simulink model "Controle_UDP_0809_simulador"  (R2014a)
settings: Solver=ode45  StartTime=0.0  StopTime=360  RelTol=1e-3
values from neighbouring files (symbols this model uses):
  Arwx = [-B1/J1 Kt/J1 ... (first row only)    [data_ACS_HIL.m]
  Arwy = [-B2/J2 Kt/J2 ... (first row only)    [data_ACS_HIL.m]
  Arwz = [-B3/J3 Kt/J3 ... (first row only)    [data_ACS_HIL.m]
  Brwx = [0 ... (first row only)    [data_ACS_HIL.m]
  Brwy = [0 ... (first row only)    [data_ACS_HIL.m]
  Brwz = [0 ... (first row only)    [data_ACS_HIL.m]
  Crwx = [1 0 ... (first row only)    [data_ACS_HIL.m]
  Crwy = [1 0 ... (first row only)    [data_ACS_HIL.m]
  Crwz = [1 0 ... (first row only)    [data_ACS_HIL.m]
  Drwx = zeros(3,1)    [data_ACS_HIL.m]
  Drwy = zeros(3,1)    [data_ACS_HIL.m]
  Drwz = zeros(3,1)    [data_ACS_HIL.m]
  I1 = 0.000624567    [data_ACS_HIL.m]
  I2 = 0.000624567    [data_ACS_HIL.m]
  I3 = 0.000624567    [data_ACS_HIL.m]
  in1 = [ 10 10 25 30 0 ] * pi / 180    [data_ACS_HIL.m]
  in2 = [ 0 10 10 30 0 ] * pi / 180    [data_ACS_HIL.m]
  in3 = [ 45 -30 30 30 0 ] * pi / 180    [data_ACS_HIL.m]
  Ixx = I( 1, 1 )    [data_ACS_HIL.m]
  Iyy = I( 2, 2 )    [data_ACS_HIL.m]
  Izz = I( 3, 3 )    [data_ACS_HIL.m]
  J1 = I1 + 3e-06    (= 0.000627567)    [data_ACS_HIL.m]
  J2 = I2 + 3e-06    (= 0.000627567)    [data_ACS_HIL.m]
  J3 = I3 + 3e-06    (= 0.000627567)    [data_ACS_HIL.m]
  Ki_x = 1    [data_ACS_HIL.m]
  Ki_y = Ki_x    (= 1)    [data_ACS_HIL.m]
  Ki_z = Ki_x    (= 1)    [data_ACS_HIL.m]
  Kp_x = 0.2    [data_ACS_HIL.m]
  Kp_y = Kp_x    (= 0.2)    [data_ACS_HIL.m]
  Kp_z = Kp_x    (= 0.2)    [data_ACS_HIL.m]
  Kpx = vp * (wn^2) * Ixx    [data_ACS_HIL.m]
  Kpy = vp * (wn^2) * Iyy    [data_ACS_HIL.m]
  Kpz = vp * (wn^2) * Izz    [data_ACS_HIL.m]
  Krx = vr * 2 * Ixx * wn * qsi    [data_ACS_HIL.m]
  Kry = vr * 2 * Iyy * wn * qsi    [data_ACS_HIL.m]
  Krz = vr * 2 * Izz * wn * qsi    [data_ACS_HIL.m]
  mW0 = 0000 / ( 60 / ( 2*pi ) )    (= 0)    [data_ACS_HIL.m]
  Wx0 = [mW0 0]    [data_ACS_HIL.m]
  Wy0 = [mW0 0]    [data_ACS_HIL.m]
  Wz0 = [mW0 0]    [data_ACS_HIL.m]
libraries: aerolibconvert2 x6, simulink x6, etargetslib x4, instrumentlib x4, aerolibutil x4, xpcutilitieslib x2, slrtlib x2, rtwinlib x1, aerolibtransform2 x1, vrlib x1
(part 1 of 2)
settings Model: Creator=mayar_000  LastModifiedBy=Toshiba Notebook
settings DataIOCC: SignalLoggingSaveFormat=ModelDataLogs
settings DebuggingCC: MultiTaskDSMMsg=warning  MultiTaskCondExecSysMsg=none  IntegerOverflowMsg=none  ParameterOverflowMsg=none
settings RTWCC: IncludeERTFirstTime=on

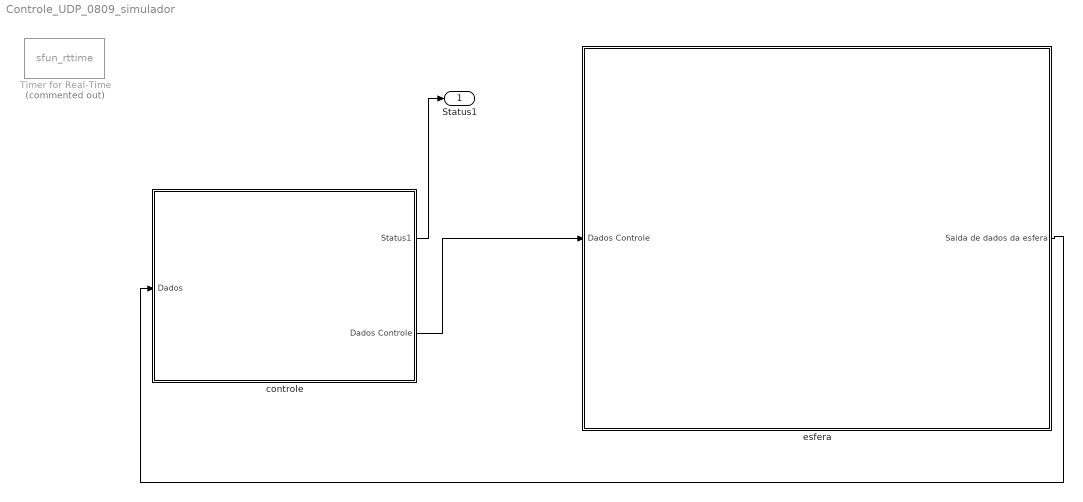
== system Controle_UDP_0809_simulador ==
  Timer for Real-Time : S-Function  Commented=on  FunctionName=sfun_rttime  Parameters=1  EnableBusSupport=off
  "controle " : Subsystem
  "esfera " : Subsystem
  Status1 : Outport
  wires:
  "controle "/1(Status1) -> Status1/1
  "esfera "/1(Saida de dados da esfera) -> "controle "/1(Dados)
  "controle "/2(Dados Controle) -> "esfera "/1(Dados Controle)

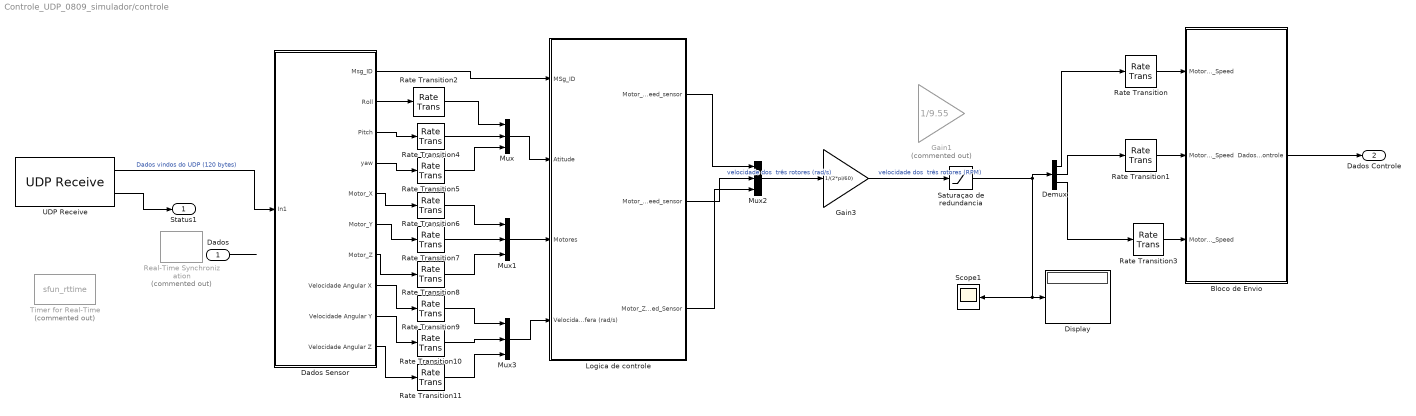
== system Controle_UDP_0809_simulador/controle  ==
  Dados : Inport
  Bloco de Envio : Subsystem
      mask Display:
      | port_label('input',1,'\Omega_x','texmode','on')
      | port_label('input',2,'\Omega_y','texmode','on')
      | port_label('input',3,'\Omega_z','texmode','on')
  Dados Sensor : Subsystem
  Demux : Demux  Outputs=3
  Display : Display
  Gain1 : Gain  Commented=on  Gain=1/9.55  SaturateOnIntegerOverflow=on
  Gain3 : Gain  Gain=1/(2*pi/60)
  Logica de controle : Subsystem
  Mux{,1..3} (4 alike) : Mux  Inputs=3
  Rate Transition{,1..5,9..11} (9 alike) : RateTransition  OutPortSampleTime=t
  Rate Transition6 : RateTransition  X0=5000  OutPortSampleTime=t
  Rate Transition7 : RateTransition  X0=5000  OutPortSampleTime=t
  Rate Transition8 : RateTransition  X0=5000  OutPortSampleTime=t
  Real-Time Synchronization : rtwinlib/Real-Time Synchronization  Commented=on  SampleTime=0.1  MaxMissedTicks=20  ShowMissedTicks=off  YieldWhenWaiting=off
  Saturaçao de redundancia : Saturate  UpperLimit=4000+mW0*60/(2*pi)  LowerLimit=-4000+mW0*60/(2*pi)
  Scope1 : Scope
      settings: YMin=-10000  YMax=10000
  Timer for Real-Time : S-Function  Commented=on  FunctionName=sfun_rttime  Parameters=1  EnableBusSupport=off
  UDP Receive : instrumentlib/UDP Receive  Host=127.0.0.1  Port=35204  LocalPort=35205  DataSize=120  EnableBlockingMode=off  Timeout=50  SampleTime=0.25  DataType=uint8  ByteOrder=BigEndian
  Status1 : Outport
  Dados Controle : Outport  Port=2  OutDataTypeStr=int16
  wires:
  UDP Receive/2 -> Status1/1
  UDP Receive/1 -> Dados Sensor/1(In1)  "Dados vindos do UDP (120 bytes)"
  Rate Transition/1 -> Bloco de Envio/1(Motor_X_Speed)
  Rate Transition1/1 -> Bloco de Envio/2(Motor_Y_Speed)
  Demux/1 -> Rate Transition/1
  Demux/2 -> Rate Transition1/1
  Demux/3 -> Rate Transition3/1
  Rate Transition3/1 -> Bloco de Envio/3(Motor_Z_Speed)
  Dados Sensor/1(Msg_ID) -> Logica de controle/1(MSg_ID)
  Mux/1 -> Logica de controle/2(Atitude)
  Mux1/1 -> Logica de controle/3(Motores)
  Logica de controle/1(Motor_X_Speed_sensor) -> Mux2/1
  Logica de controle/2(Motor_Y_Speed_sensor) -> Mux2/2
  Logica de controle/3(Motor_Z_Speed_Sensor) -> Mux2/3
  Dados Sensor/2(Roll) -> Rate Transition2/1
  Dados Sensor/3(Pitch) -> Rate Transition4/1
  Dados Sensor/4(yaw) -> Rate Transition5/1
  Dados Sensor/7(Motor_Z) -> Rate Transition8/1
  Dados Sensor/6(Motor_Y) -> Rate Transition7/1
  Dados Sensor/5(Motor_X) -> Rate Transition6/1
  Rate Transition2/1 -> Mux/1
  Rate Transition4/1 -> Mux/2
  Rate Transition5/1 -> Mux/3
  Rate Transition6/1 -> Mux1/1
  Rate Transition7/1 -> Mux1/2
  Rate Transition8/1 -> Mux1/3
  Saturaçao de redundancia/1 -> Demux/1, Scope1/1, Display/1
  Mux2/1 -> Gain3/1  "velocidade dos  três rotores (rad/s)"
  Gain3/1 -> Saturaçao de redundancia/1  "velocidade dos  três rotores (RPM)"
  Dados Sensor/8(Velocidade Angular X) -> Rate Transition9/1
  Dados Sensor/9(Velocidade Angular Y) -> Rate Transition10/1
  Dados Sensor/10(Velocidade Angular Z) -> Rate Transition11/1
  Mux3/1 -> Logica de controle/4(Velocidade Angular da Esfera (rad/s))
  Rate Transition9/1 -> Mux3/1
  Rate Transition10/1 -> Mux3/2
  Rate Transition11/1 -> Mux3/3
  Dados/1 -> ?
  Bloco de Envio/1(Dados Controle) -> Dados Controle/1

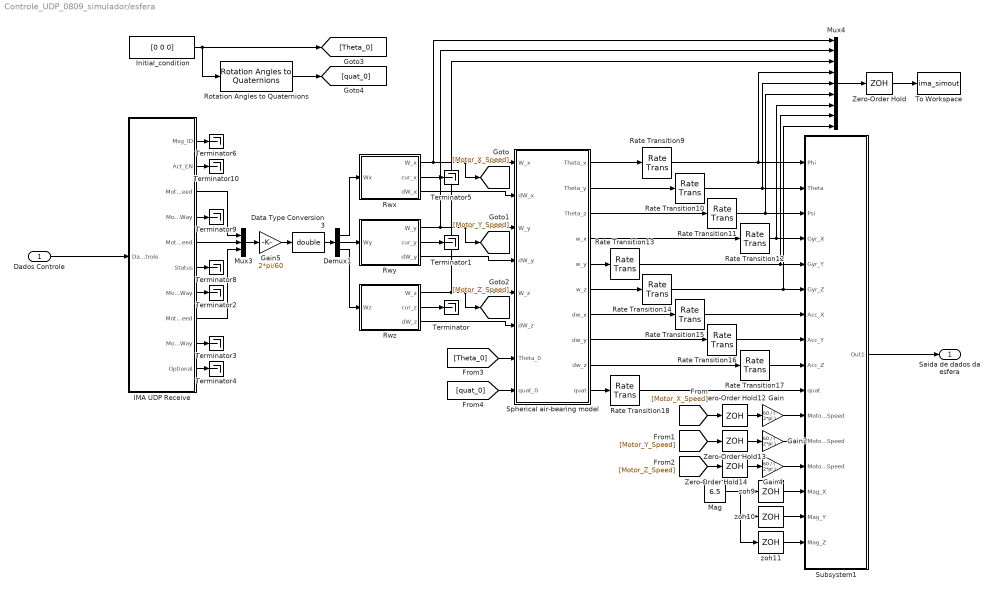
== system Controle_UDP_0809_simulador/esfera  ==
  Dados Controle : Inport
  Data Type Conversion3 : DataTypeConversion  OutDataTypeStr=double  SaturateOnIntegerOverflow=on
  Demux1 : Demux  Outputs=3
  Gain : Gain  Gain=60 / ( 2*pi )
  Gain2 : Gain  Gain=60 / ( 2*pi )
  Gain4 : Gain  Gain=60 / ( 2*pi )
  Gain5 : Gain  Gain=2*pi/60
  IMA UDP Receive : Subsystem
  Initial_condition : Constant  Value=[0 0 0]
  Mag : Constant  Value=6.5  OutDataTypeStr=single
  Mux3 : Mux  Inputs=3
  Mux4 : Mux  Inputs=9
  Rate Transition{9..18} (10 alike) : RateTransition  OutPortSampleTime=t
  Rotation Angles to Quaternions : aerolibtransform2/Rotation Angles to Quaternions  rotationOrder=XYZ
  Rwx : Subsystem
      mask Display:
      | port_label('input',1,'\Omega_{x}^{ref}','texmode','on')
      | 
      | 
      | port_label('output',1,'\Omega_{x}','texmode','on')
      | port_label('output',2,'i_{x}','texmode','on')
      | port_label('output',3,'d\Omega_{x}','texmode','on')
  Rwy : Subsystem
      mask Display:
      | port_label('input',1,'\Omega_{y}^{ref}','texmode','on')
      | 
      | port_label('output',1,'\Omega_{y}','texmode','on')
      | port_label('output',2,'i_{y}','texmode','on')
      | port_label('output',3,'d\Omega_{y}','texmode','on')
  Rwz : Subsystem
      mask Display:
      | port_label('input',1,'\Omega_{z}^{ref}','texmode','on')
      | 
      | port_label('output',1,'\Omega_{z}','texmode','on')
      | port_label('output',2,'i_{z}','texmode','on')
      | port_label('output',3,'d\Omega_{z}','texmode','on')
  Spherical air-bearing model : Subsystem
      mask Display:
      | port_label('input',1,'\Omega_x','texmode','on')
      | port_label('input',2,'d\Omega_x','texmode','on')
      | port_label('input',3,'\Omega_y','texmode','on')
      | port_label('input',4,'d\Omega_y','texmode','on')
      | port_label('input',5,'\Omega_z','texmode','on')
      | port_label('input',6,'d\Omega_z','texmode','on')
      | port_label('input',7,'\theta_{0}','texmode','on')
      | port_label('input',8,'q_{0}','texmode','on')
      | 
      | port_label('output',1,'\theta_x','texmode','on')
      | port_label('output',2,'\theta_y','texmode','on')
      | port_label('output',3,'\theta_z','texmode','on')
      | port_label('output',4,'\omega_x','texmode','on')
      | port_label('output',5,'\omega_y','texmode','on')
      | port_label('output',6,'\omega_z','texmode','on')
      | port_label('output',7,'d\omega_x','texmode','on')
      | port_label('output',8,'d\omega_y','texmode','on')
      | port_label('output',9,'d\omega_z','texmode','on')
      | port_label('output',10,'q','texmode','on')
  Subsystem1 : Subsystem
      mask Display:
      | port_label('input',1,'\theta_x','texmode','on')
      | port_label('input',2,'\theta_y','texmode','on')
      | port_label('input',3,'\theta_z','texmode','on')
      | port_label('input',4,'\omega_x','texmode','on')
      | port_label('input',5,'\omega_y','texmode','on')
      | port_label('input',6,'\omega_z','texmode','on')
      | port_label('input',7,'d\omega_x','texmode','on')
      | port_label('input',8,'d\omega_y','texmode','on')
      | port_label('input',9,'d\omega_z','texmode','on')
      | port_label('input',10,'q','texmode','on')
      | port_label('input',11,'\Omega_x','texmode','on')
      | port_label('input',12,'\Omega_y','texmode','on')
      | port_label('input',13,'\Omega_z','texmode','on')
      | port_label('input',14,'B_x','texmode','on')
      | port_label('input',15,'B_y','texmode','on')
      | port_label('input',16,'B_z','texmode','on')
  Terminator{,1..6,8..10} (10 alike) : Terminator
  To Workspace : ToWorkspace  VariableName=ima_simout  SampleTime=-1
  Zero-Order Hold : ZeroOrderHold  SampleTime=0.5
  Zero-Order Hold12 : ZeroOrderHold  SampleTime=t
  Zero-Order Hold13 : ZeroOrderHold  SampleTime=t
  Zero-Order Hold14 : ZeroOrderHold  SampleTime=t
  zoh10 : ZeroOrderHold  SampleTime=t
  zoh11 : ZeroOrderHold  SampleTime=t
  zoh9 : ZeroOrderHold  SampleTime=t
  Saida de dados da esfera : Outport
  wires:
  Rate Transition12/1 -> Subsystem1/4(Gyr_X), Mux4/7
  Spherical air-bearing model/2(Theta_y) -> Rate Transition10/1
  Initial_condition/1 -> [Theta_0], Rotation Angles to Quaternions/1
  Rwy/2(cur_y) -> Terminator1/1
  Rate Transition16/1 -> Subsystem1/8(Acc_Y)
  IMA UDP Receive/7(Motor_Y_Way) -> Terminator2/1
  IMA UDP Receive/9(Motor_Z_Way) -> Terminator3/1
  Data Type Conversion3/1 -> Demux1/1
  Spherical air-bearing model/4(w_x) -> Rate Transition12/1
  IMA UDP Receive/4(Motor_X_Way) -> Terminator9/1
  Spherical air-bearing model/3(Theta_z) -> Rate Transition11/1
  IMA UDP Receive/5(Motor_Y_Speed) -> Mux3/2
  IMA UDP Receive/10(Optional) -> Terminator4/1
  Rate Transition17/1 -> Subsystem1/9(Acc_Z)
  zoh9/1 -> Subsystem1/14(Mag_X)
  Spherical air-bearing model/6(w_z) -> Rate Transition14/1
  Rate Transition11/1 -> Subsystem1/3(Psi), Mux4/6
  Spherical air-bearing model/8(dw_y) -> Rate Transition16/1
  Rate Transition10/1 -> Subsystem1/2(Theta), Mux4/5
  Spherical air-bearing model/7(dw_x) -> Rate Transition15/1
  Demux1/2 -> Rwy/1(Wy)
  Demux1/3 -> Rwz/1(Wz)
  Rate Transition9/1 -> Subsystem1/1(Phi), Mux4/4
  Rate Transition15/1 -> Subsystem1/7(Acc_X)
  zoh11/1 -> Subsystem1/16(Mag_Z)
  zoh10/1 -> Subsystem1/15(Mag_Y)
  Spherical air-bearing model/9(dw_z) -> Rate Transition17/1
  Rwz/2(cur_z) -> Terminator/1
  IMA UDP Receive/1(Msg_ID) -> Terminator6/1
  IMA UDP Receive/6(Status) -> Terminator8/1
  IMA UDP Receive/2(Act_EN) -> Terminator10/1
  Rate Transition13/1 -> Subsystem1/5(Gyr_Y), Mux4/8
  Demux1/1 -> Rwx/1(Wx)
  Spherical air-bearing model/1(Theta_x) -> Rate Transition9/1
  Rate Transition14/1 -> Subsystem1/6(Gyr_Z), Mux4/9
  Spherical air-bearing model/5(w_y) -> Rate Transition13/1
  [Theta_0] -> Spherical air-bearing model/7(Theta_0)
  Mux3/1 -> Gain5/1
  Spherical air-bearing model/10(quat) -> Rate Transition18/1
  Rwz/1(W_z) -> Spherical air-bearing model/5(W_z), [Motor_Z_Speed], Mux4/3
  Gain/1 -> Subsystem1/11(Motor_X_Speed)
  [Motor_X_Speed] -> Zero-Order Hold12/1
  IMA UDP Receive/8(Motor_Z_Speed) -> Mux3/3
  Zero-Order Hold14/1 -> Gain4/1
  Rwx/2(cur_x) -> Terminator5/1
  IMA UDP Receive/3(Motor_X_Speed) -> Mux3/1
  Gain5/1 -> Data Type Conversion3/1
  Gain2/1 -> Subsystem1/12(Motor_Y_Speed)
  Mag/1 -> zoh9/1, zoh10/1, zoh11/1
  [Motor_Y_Speed] -> Zero-Order Hold13/1
  Gain4/1 -> Subsystem1/13(Motor_Z_Speed)
  [Motor_Z_Speed] -> Zero-Order Hold14/1
  Zero-Order Hold12/1 -> Gain/1
  [quat_0] -> Spherical air-bearing model/8(quat_0)
  Rotation Angles to Quaternions/1 -> [quat_0]
  Zero-Order Hold13/1 -> Gain2/1
  Rwx/1(W_x) -> Spherical air-bearing model/1(W_x), [Motor_X_Speed], Mux4/1
  Rwz/3(dW_z) -> Spherical air-bearing model/6(dW_z)
  Zero-Order Hold/1 -> To Workspace/1
  Rate Transition18/1 -> Subsystem1/10(quat)
  Rwy/1(W_y) -> Spherical air-bearing model/3(W_y), [Motor_Y_Speed], Mux4/2
  Rwx/3(dW_x) -> Spherical air-bearing model/2(dW_x)
  Rwy/3(dW_y) -> Spherical air-bearing model/4(dW_y)
  Mux4/1 -> Zero-Order Hold/1
  Subsystem1/1(Out1) -> Saida de dados da esfera/1
  Dados Controle/1 -> IMA UDP Receive/1(Dados Controle)

== system Controle_UDP_0809_simulador/controle /Bloco de Envio ==
  Motor_X_Speed : Inport
  Motor_Y_Speed : Inport  Port=2
  Motor_Z_Speed : Inport  Port=3
  "Byte Packing " : xpcutilitieslib/Byte Packing   MaskPackedDataType=uint8  MaskUnpackedDataTypes={'uint8','uint8','int16','uint8','int16','uint8','int16','uint8', 'uint8'}  MaskAlignment=1
  Byte Reversal3 : etargetslib/Byte Reversal  numInp=3
  Data Type Conversion17 : DataTypeConversion  OutDataTypeStr=int16  SaturateOnIntegerOverflow=on
  Data Type Conversion2 : DataTypeConversion  OutDataTypeStr=uint8  SaturateOnIntegerOverflow=on
  Data Type Conversion6 : DataTypeConversion  OutDataTypeStr=int16  SaturateOnIntegerOverflow=on
  Data Type Conversion8 : DataTypeConversion  OutDataTypeStr=int16  SaturateOnIntegerOverflow=on
  Display{1..4} (4 alike) : Display
      Display3 settings: Format=hex (Stored Integer)
      Display4 settings: Format=hex (Stored Integer)
  ID1 : Constant  OutDataTypeStr=uint8
  Mux1 : Mux  Inputs=3
  Mux2 : Mux  Inputs=3
  Mux3 : Mux  Inputs=3
  UDP Send1 : instrumentlib/UDP Send  Host=127.0.0.1  Port=35207  LocalPort=35206  EnableBlockingMode=off  ByteOrder=LittleEndian
  Dados Controle : Outport  OutDataTypeStr=int16
  wires:
  Motor_Y_Speed/1 -> Mux3/2, Data Type Conversion8/1
  Data Type Conversion6/1 -> Mux2/1, Byte Reversal3/1
  Motor_X_Speed/1 -> Mux3/1, Data Type Conversion6/1
  "Byte Packing "/1 -> UDP Send1/1, Display2/1
  Data Type Conversion8/1 -> Mux2/2, Byte Reversal3/2
  Data Type Conversion17/1 -> Mux2/3, Byte Reversal3/3
  Byte Reversal3/2 -> Mux1/2, "Byte Packing "/5
  Data Type Conversion2/1 -> "Byte Packing "/9, "Byte Packing "/8, "Byte Packing "/6, "Byte Packing "/4, "Byte Packing "/2, "Byte Packing "/1
  ID1/1 -> Data Type Conversion2/1
  Byte Reversal3/1 -> Mux1/1, "Byte Packing "/3
  Mux3/1 -> Display1/1
  Mux1/1 -> Display4/1
  Byte Reversal3/3 -> Mux1/3, "Byte Packing "/7
  Motor_Z_Speed/1 -> Mux3/3, Data Type Conversion17/1
  Mux2/1 -> Display3/1

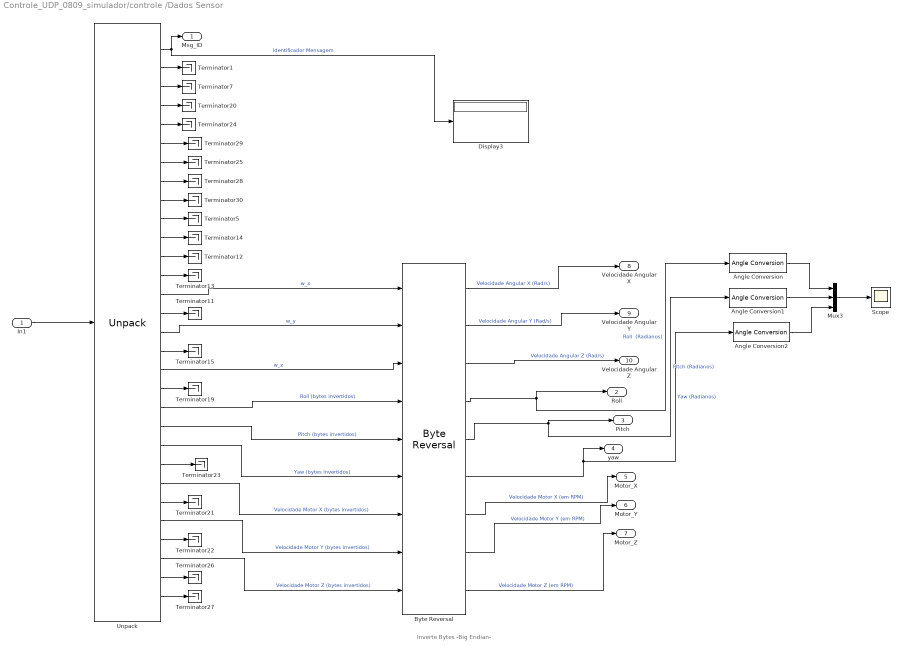
== system Controle_UDP_0809_simulador/controle /Dados Sensor ==
  note: Inverte Bytes
      | -Big Endian-
  In1 : Inport
  Angle Conversion : aerolibconvert2/Angle Conversion  IU=rad  OU=deg
  Angle Conversion1 : aerolibconvert2/Angle Conversion  IU=rad  OU=deg
  Angle Conversion2 : aerolibconvert2/Angle Conversion  IU=rad  OU=deg
  Byte Reversal : etargetslib/Byte Reversal  numInp=9
  Display3 : Display
  Mux3 : Mux  Inputs=3
  Scope : Scope
      settings: YMin=0.2  YMax=1.5  SaveName=ScopeData2
  Terminator{1,5,7,11..15,19..30} (20 alike) : Terminator
  Unpack : slrtlib/UDP/Unpack   dimensions={[1,1],[1,1],[1,1],[1,1],[1,1],[1,1],[1,1],[1,1],[1,1],[1,1],[1,1],[1,1],[1,1],[1,1],[1,1],[1,1],[1,1],[1,1],[1,1],[1,1],[1,1],[1,1],[1,4],[1,1],[1,1],[1,1],[1,1],[1,1],[1,1],[1,1]}  datatypes={'uint8','single','uint32','single','uint32','single','uint32','single','uint32','single','uint32','single','uint32','single','uint32','single','uint32','single','uint32','single','single','single','single','int16','uint32','int16','uint32','int16','uint32','uint8'}  byteAlign=1
  Msg_ID : Outport
  Roll : Outport  Port=2
  Pitch : Outport  Port=3
  yaw : Outport  Port=4
  Motor_X : Outport  Port=5
  Motor_Y : Outport  Port=6
  Motor_Z : Outport  Port=7
  Velocidade Angular X : Outport  Port=8
  Velocidade Angular Y : Outport  Port=9
  Velocidade Angular Z : Outport  Port=10
  wires:
  Unpack/4 -> Terminator20/1
  Unpack/5 -> Terminator24/1
  Unpack/6 -> Terminator29/1
  Unpack/3 -> Terminator7/1
  Byte Reversal/8 -> Motor_Y/1  "Velocidade Motor Y (em RPM)"
  Unpack/1 -> Msg_ID/1, Display3/1  "Identificador Mensagem"
  Unpack/2 -> Terminator1/1
  Unpack/7 -> Terminator25/1
  Unpack/8 -> Terminator28/1
  Byte Reversal/5 -> Pitch/1, Angle Conversion1/1  "Pitch (Radianos)"
  Byte Reversal/7 -> Motor_X/1  "Velocidade Motor X (em RPM)"
  Unpack/28 -> Byte Reversal/9  "Velocidade Motor Z (bytes invertidos)"
  Unpack/19 -> Terminator19/1
  Unpack/11 -> Terminator14/1
  Unpack/14 -> Byte Reversal/1  "w_x"
  Unpack/16 -> Byte Reversal/2  "w_y"
  Unpack/30 -> Terminator27/1
  Unpack/20 -> Byte Reversal/4  "Roll (bytes invertidos)"
  Unpack/21 -> Byte Reversal/5  "Pitch (bytes invertidos)"
  Unpack/12 -> Terminator12/1
  Unpack/23 -> Terminator23/1
  Unpack/18 -> Byte Reversal/3  "w_z"
  Unpack/27 -> Terminator22/1
  Unpack/25 -> Terminator21/1
  Unpack/15 -> Terminator11/1
  Unpack/13 -> Terminator13/1
  Unpack/10 -> Terminator5/1
  Unpack/9 -> Terminator30/1
  Unpack/17 -> Terminator15/1
  Unpack/22 -> Byte Reversal/6  "Yaw (bytes invertidos)"
  Unpack/24 -> Byte Reversal/7  "Velocidade Motor X (bytes invertidos)"
  Unpack/26 -> Byte Reversal/8  "Velocidade Motor Y (bytes invertidos)"
  Unpack/29 -> Terminator26/1
  Byte Reversal/4 -> Roll/1, Angle Conversion/1  "Roll  (Radianos)"
  Byte Reversal/9 -> Motor_Z/1  "Velocidade Motor Z (em RPM)"
  Byte Reversal/6 -> yaw/1, Angle Conversion2/1  "Yaw (Radianos)"
  In1/1 -> Unpack/1
  Angle Conversion/1 -> Mux3/1
  Angle Conversion1/1 -> Mux3/2
  Angle Conversion2/1 -> Mux3/3
  Mux3/1 -> Scope/1
  Byte Reversal/3 -> Velocidade Angular Z/1  "Velocidade Angular Z (Rad/s)"
  Byte Reversal/2 -> Velocidade Angular Y/1  "Velocidade Angular Y (Rad/s)"
  Byte Reversal/1 -> Velocidade Angular X/1  "Velocidade Angular X (Rad/s)"

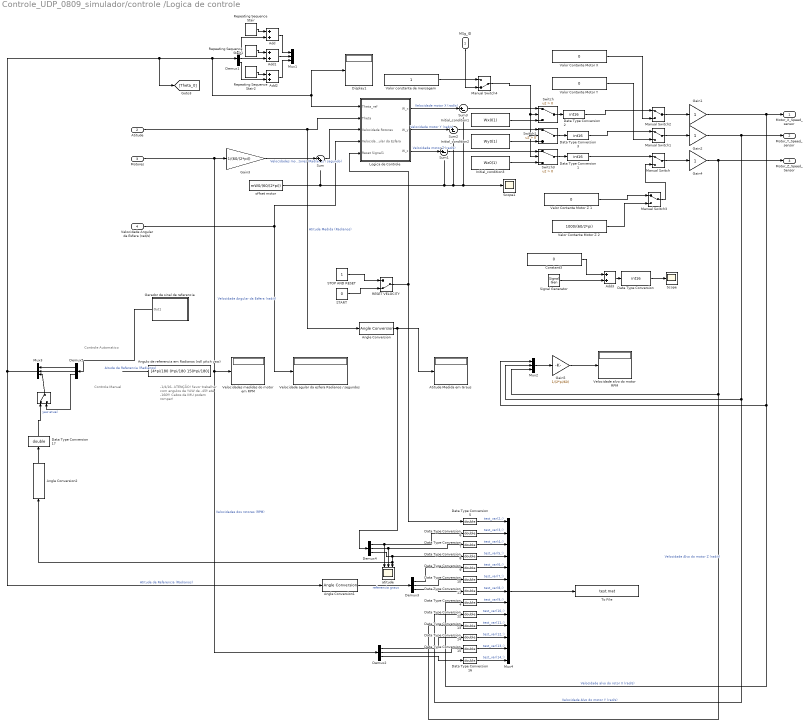
== system Controle_UDP_0809_simulador/controle /Logica de controle ==
  note: Controle Automatico
  note: Controle Manual
  note: -1/4/16-
      | ATENÇÃO!
      |
      | favor trabalhar com
      | angulos de YAW de
      | -45º até -160º!
      | Cabos da IMU podem romper!
  MSg_ID : Inport
  Atitude : Inport  Port=2
  Motores : Inport  Port=3
  Velocidade Angular da Esfera (rad/s) : Inport  Port=4
  " " : ManualSwitch
  Add{,1..3} (4 alike) : Sum
  Angle Conversion : aerolibconvert2/Angle Conversion  IU=rad  OU=deg
  Angle Conversion1 : aerolibconvert2/Angle Conversion  IU=rad  OU=deg
  Angle Conversion2 : aerolibconvert2/Angle Conversion  IU=deg  OU=rad
  Angulo de referencia em Radianos (roll pitch yaw) : Constant  Value=[4*pi/180 0*pi/180 150*pi/180]  VectorParams1D=off
  Atitude Medida em Graus : Display
      settings: Decimation=3
  Constant3 : Constant  Value=0  OutDataTypeStr=int16
  Data Type Conversion : DataTypeConversion  OutDataTypeStr=int16
  Data Type Conversion1 : DataTypeConversion  OutDataTypeStr=int16  SaturateOnIntegerOverflow=on
  Data Type Conversion{4..17} (14 alike) : DataTypeConversion  OutDataTypeStr=double  SaturateOnIntegerOverflow=on
  Data Type Conversion2 : DataTypeConversion  OutDataTypeStr=int16  SaturateOnIntegerOverflow=on
  Data Type Conversion3 : DataTypeConversion  OutDataTypeStr=int16  SaturateOnIntegerOverflow=on
  Demux{1..5} (5 alike) : Demux  Outputs=3
  Display1 : Display
  Gain1 : Gain  OutDataTypeStr=int16  SaturateOnIntegerOverflow=on
  Gain2 : Gain  OutDataTypeStr=int16  SaturateOnIntegerOverflow=on
  Gain3 : Gain  Gain=1/(60/(2*pi))
  Gain4 : Gain  OutDataTypeStr=int16  SaturateOnIntegerOverflow=on
  Gain5 : Gain  Gain=1/(2*pi/60)  OutDataTypeStr=int16  SaturateOnIntegerOverflow=on
  Gerador de sinal de referencia : Subsystem
  Initial_condition1 : Constant  Value=Wx0(1)  OutDataTypeStr=int16
  Initial_condition2 : Constant  Value=Wy0(1)  OutDataTypeStr=int16
  Initial_condition3 : Constant  Value=Wz0(1)  OutDataTypeStr=int16
  Logica de Controle : Subsystem
      mask Display:
      | port_label('input',1,'\theta^{ref}','texmode','on')
      | port_label('input',2,'\theta','texmode','on')
      | port_label('input',3,'\Omega','texmode','on')
      | port_label('input',4,'\omega','texmode','on')
      | port_label('input',5,'RESET','texmode','on')
      | 
      | port_label('output',1,'\Omega_{x}^{des}','texmode','on')
      | port_label('output',2,'\Omega_{y}^{des}','texmode','on')
      | port_label('output',3,'\Omega_{z}^{des}','texmode','on')
  Manual Switch{,1..3} (4 alike) : ManualSwitch
  Manual Switch4 : ManualSwitch  CurrentSetting=0
  Mux1 : Mux  Inputs=3
  Mux2 : Mux  Inputs=3
  Mux3 : Mux  Inputs=3
  Mux4 : Mux  Inputs=13
  RESET VELOCITY : ManualSwitch  CurrentSetting=0
  Repeating Sequence Stair : simulink/Sources/Repeating Sequence Stair  OutValues=in1.'  tsamp=1000  OutMin=[]  OutMax=[]  OutDataTypeStr=double  OutputDataTypeScalingMode=double  OutDataType=fixdt(0,8)  ConRadixGroup=Best Precision: Vector-wise  OutScaling=2^-12
  Repeating Sequence Stair1 : simulink/Sources/Repeating Sequence Stair  OutValues=in2.'  tsamp=1000  OutMin=[]  OutMax=[]  OutDataTypeStr=double  OutputDataTypeScalingMode=double  OutDataType=fixdt(0,8)  ConRadixGroup=Best Precision: Vector-wise  OutScaling=2^-12
  Repeating Sequence Stair2 : simulink/Sources/Repeating Sequence Stair  OutValues=in3.'  tsamp=1000  OutMin=[]  OutMax=[]  OutDataTypeStr=double  OutputDataTypeScalingMode=double  OutDataType=fixdt(0,8)  ConRadixGroup=Best Precision: Vector-wise  OutScaling=2^-12
  START : Constant  Value=0  OutDataTypeStr=boolean
  STOP AND RESET : Constant  OutDataTypeStr=boolean
  Scope : Scope
      settings: YMin=-1050  YMax=-950  SaveName=sinal_referencia
  Scope1 : Scope
      settings: YMin=523.599  YMax=523.599  SaveName=sinal_referencia1
  Signal Generator : SignalGenerator  WaveForm=square  Amplitude=1000  Frequency=0.1
  Sum : Sum  Inputs=|++
  Sum1 : Sum  Inputs=|+-
  Sum2 : Sum  Inputs=|+-
  Sum3 : Sum  Inputs=|+-
  Switch : Switch  Criteria=u2 > Threshold  OutDataTypeStr=int16
  Switch1 : Switch  Criteria=u2 > Threshold  OutDataTypeStr=int16
  Switch3 : Switch  Criteria=u2 > Threshold  OutDataTypeStr=int16
  To File : ToFile  Filename=test.mat  MatrixName=test_var
  Valor Contante Motor X : Constant  Value=0  OutDataTypeStr=int16
  Valor Contante Motor Y : Constant  Value=0  OutDataTypeStr=int16
  Valor Contante Motor Z 1 : Constant  Value=0  OutDataTypeStr=int16
  Valor Contante Motor Z 2 : Constant  Value=1000/(60/2*pi)  OutDataTypeStr=int16
  Valor constante de mensagem : Constant  OutDataTypeStr=int16
  Velocidade agular da esfera Radianos / segundos : Display
      settings: Format=decimal (Stored Integer)  Decimation=3
  Velocidade alvo do motor RPM : Display
      settings: Decimation=3
  Velocidades medidas do motor em RPM : Display
      settings: Decimation=3
  atitude : Scope  NumInputPorts=3
      settings: YMin=3.86202~0.75~-0.5  YMax=3.86202~3~2.25  SaveName=ScopeData4
  offset motor : Constant  Value=mW0/(60/(2*pi))  OutDataTypeStr=double
  Motor_X_Speed_sensor : Outport
  Motor_Y_Speed_sensor : Outport  Port=2
  Motor_Z_Speed_Sensor : Outport  Port=3  OutDataTypeStr=int16
  wires:
  Add1/1 -> Mux1/2
  Demux1/1 -> Add/2
  Add2/1 -> Mux1/3
  Mux3/1 -> Logica de Controle/1(Theta_ref), Display1/1, Demux1/1, [Theta_0], Angle Conversion1/1  "Atitude de Referencia (Radianos)"
  Demux1/2 -> Add1/2
  Repeating Sequence Stair/1 -> Add/1
  Repeating Sequence Stair2/1 -> Add2/1
  Repeating Sequence Stair1/1 -> Add1/1
  Demux1/3 -> Add2/2
  Add/1 -> Mux1/1
  Initial_condition1/1 -> Switch/3
  Motores/1 -> Demux2/1, Velocidades medidas do motor em RPM/1, Gain3/1  "Velocidades dos rotores (RPM)"
  Initial_condition2/1 -> Switch1/3
  Logica de Controle/1(W_x) -> Sum3/1  "Velocidade motor X (rad/s)"
  Logica de Controle/2(W_y) -> Sum2/1  "Velocidade motor Y (rad/s)"
  Logica de Controle/3(W_z) -> Sum1/1  "Velocidade motor Z (rad/s)"
  Switch/1 -> Data Type Conversion2/1
  Data Type Conversion/1 -> Scope/1
  Initial_condition3/1 -> Switch3/3
  Signal Generator/1 -> Add3/2
  Constant3/1 -> Add3/1
  Add3/1 -> Data Type Conversion/1
  Switch3/1 -> Data Type Conversion1/1
  Switch1/1 -> Data Type Conversion3/1
  Valor Contante Motor Y/1 -> Manual Switch1/2
  Valor Contante Motor X/1 -> Manual Switch2/2
  Gain3/1 -> Sum/1  "Velocidades motores (Radianos / segundo)"
  Manual Switch/1 -> Gain4/1
  Manual Switch1/1 -> Gain2/1
  Manual Switch2/1 -> Gain1/1
  Gain1/1 -> Data Type Conversion4/1, Mux2/1, Motor_X_Speed_sensor/1  "Velocidade alvo do rotor X (rad/s)"
  Gain2/1 -> Mux2/2, Data Type Conversion12/1, Motor_Y_Speed_sensor/1  "Velocidade Alvo do motor Y (rad/s)"
  Gain4/1 -> Data Type Conversion13/1, Mux2/3, Motor_Z_Speed_Sensor/1  "Velocidade Alvo do motor Z (rad/s)"
  Atitude/1 -> Logica de Controle/2(Theta), Angle Conversion/1  "Atitude Medida (Radianos)"
  Valor Contante Motor Z 1/1 -> Manual Switch3/1
  Valor Contante Motor Z 2/1 -> Manual Switch3/2
  Manual Switch3/1 -> Manual Switch/2
  Valor constante de mensagem/1 -> Manual Switch4/1
  MSg_ID/1 -> Manual Switch4/2
  Manual Switch4/1 -> Switch3/2, Switch1/2, Switch/2
  STOP AND RESET/1 -> RESET VELOCITY/1
  START/1 -> RESET VELOCITY/2
  Mux2/1 -> Gain5/1
  Gain5/1 -> Velocidade alvo do motor RPM/1
  Sum/1 -> Logica de Controle/3(Velocidade Rotores)
  Velocidade Angular da Esfera (rad/s)/1 -> Logica de Controle/4(Velocidade Angular da Esfera), Velocidade agular da esfera Radianos / segundos/1  "Velocidade Angular da Esfera (rad/s)"
  Angle Conversion/1 -> Demux4/1, Atitude Medida em Graus/1
  Mux4/1 -> To File/1
  RESET VELOCITY/1 -> Data Type Conversion5/1, Logica de Controle/5(Reset Signal1)
  Demux4/2 -> Data Type Conversion7/1, atitude/2
  Demux4/1 -> Data Type Conversion6/1, atitude/1
  Data Type Conversion5/1 -> Mux4/1  "test_var(2,:)"
  Data Type Conversion6/1 -> Mux4/2  "test_var(3,:)"
  Data Type Conversion7/1 -> Mux4/3  "test_var(4,:)"
  Data Type Conversion8/1 -> Mux4/4  "test_var(5,:)"
  Data Type Conversion9/1 -> Mux4/5  "test_var(6,:)"
  Data Type Conversion10/1 -> Mux4/6  "test_var(7,:)"
  Data Type Conversion11/1 -> Mux4/7  "test_var(8,:)"
  Data Type Conversion4/1 -> Mux4/8  "test_var(9,:)"
  Data Type Conversion14/1 -> Mux4/11  "test_var(12,:)"
  Data Type Conversion15/1 -> Mux4/12  "test_var(13,:)"
  Data Type Conversion13/1 -> Mux4/10  "test_var(11,:)"
  Data Type Conversion12/1 -> Mux4/9  "test_var(10,:)"
  Data Type Conversion16/1 -> Mux4/13  "test_var(14,:)"
  Demux2/3 -> Data Type Conversion16/1
  Demux2/1 -> Data Type Conversion14/1
  Demux2/2 -> Data Type Conversion15/1
  Demux3/3 -> Data Type Conversion11/1
  Demux3/2 -> Data Type Conversion10/1
  Demux3/1 -> Data Type Conversion9/1
  Angle Conversion1/1 -> Demux3/1  "referencia graus"
  Demux5/1 -> Mux3/1
  Demux5/2 -> Mux3/2
  Demux4/3 -> Data Type Conversion8/1, Angle Conversion2/1, atitude/3
  Data Type Conversion17/1 -> " "/1  "yaw atual"
  " "/1 -> Mux3/3
  Demux5/3 -> " "/2
  Angle Conversion2/1 -> Data Type Conversion17/1
  Gerador de sinal de referencia/1(Out1) -> Demux5/1
  Angulo de referencia em Radianos (roll pitch yaw)/1 -> ?  "Aitude de Referencia (Radianos)"
  Sum3/1 -> Switch/1
  Sum2/1 -> Switch1/1
  Sum1/1 -> Switch3/1
  Data Type Conversion1/1 -> Manual Switch/1
  Data Type Conversion3/1 -> Manual Switch1/1
  Data Type Conversion2/1 -> Manual Switch2/1
  offset motor/1 -> Scope1/1

== system Controle_UDP_0809_simulador/esfera /IMA UDP Receive ==
  Dados Controle : Inport
  Byte Reversal : etargetslib/Byte Reversal  numInp=3
  Initial_condition : Constant  Value=Wx0(1) * 60 / ( 2*pi )
  Initial_condition1 : Constant  Value=Wy0(1) * 60 / ( 2*pi )
  Initial_condition2 : Constant  Value=Wz0(1) * 60 / ( 2*pi )
  Switch : Switch  Criteria=u2 > Threshold
  Switch1 : Switch  Criteria=u2 > Threshold
  Switch2 : Switch  Criteria=u2 > Threshold
  UDP Receive : instrumentlib/UDP Receive  Host=127.0.0.1  Port=35206  LocalPort=35207  DataSize=12  EnableBlockingMode=off  Timeout=50  SampleTime=0.25  DataType=uint8  ByteOrder=BigEndian
  Unpack1 : slrtlib/UDP/Unpack   dimensions={[1,1],[1,1],[1,1],[1,1],[1,1],[1,1],[1,1],[1,1],[1,1]}  datatypes={'uint8','uint8','int16','uint8','int16','uint8','int16','uint8', 'uint8'}  byteAlign=1
  Msg_ID : Outport
  Act_EN : Outport  Port=2
  Motor_X_Speed : Outport  Port=3
  Motor_X_Way : Outport  Port=4
  Motor_Y_Speed : Outport  Port=5
  Status : Outport  Port=6
  Motor_Y_Way : Outport  Port=7
  Motor_Z_Speed : Outport  Port=8
  Motor_Z_Way : Outport  Port=9
  Optional : Outport  Port=10
  wires:
  Unpack1/9 -> Optional/1
  Unpack1/8 -> Motor_Z_Way/1
  Unpack1/6 -> Motor_Y_Way/1
  Unpack1/4 -> Motor_X_Way/1
  Unpack1/2 -> Act_EN/1
  Unpack1/1 -> Msg_ID/1, Switch1/2, Switch2/2, Switch/2
  Unpack1/3 -> Byte Reversal/1
  Unpack1/5 -> Byte Reversal/2
  Unpack1/7 -> Byte Reversal/3
  UDP Receive/2 -> Status/1
  UDP Receive/1 -> Unpack1/1
  Initial_condition/1 -> Switch/3
  Switch/1 -> Motor_X_Speed/1
  Initial_condition1/1 -> Switch1/3
  Switch1/1 -> Motor_Y_Speed/1
  Initial_condition2/1 -> Switch2/3
  Switch2/1 -> Motor_Z_Speed/1
  Byte Reversal/3 -> Switch2/1
  Byte Reversal/2 -> Switch1/1
  Byte Reversal/1 -> Switch/1
  Dados Controle/1 -> ?

== system Controle_UDP_0809_simulador/esfera /Rwx ==
  Wx : Inport
  Demux : Demux  Outputs=3
  Integrator : Integrator  InitialCondition=Wx0(1)/47.149
  Ki_x : Gain  Gain=Ki_x
  Kp_x : Gain  Gain=Kp_x
  Motor_Rwx : StateSpace  A=Arwx  B=Brwx  C=Crwx  D=Drwx  X0=Wx0
  Saturation : Saturate  UpperLimit=100  LowerLimit=-100
  Sum : Sum  Inputs=|+-
  Sum1 : Sum  Inputs=|++
  W_x : Outport
  cur_x : Outport  Port=2
  dW_x : Outport  Port=3
  wires:
  Sum/1 -> Kp_x/1, Ki_x/1
  Ki_x/1 -> Integrator/1
  Integrator/1 -> Sum1/2
  Kp_x/1 -> Sum1/1
  Sum1/1 -> Saturation/1
  Motor_Rwx/1 -> Demux/1
  Demux/3 -> dW_x/1
  Demux/1 -> Sum/2, W_x/1
  Saturation/1 -> Motor_Rwx/1
  Demux/2 -> cur_x/1
  Wx/1 -> Sum/1

== system Controle_UDP_0809_simulador/esfera /Rwy ==
  Wy : Inport
  Demux : Demux  Outputs=3
  Integrator : Integrator  InitialCondition=Wy0(1)/47.149
  Ki_y : Gain  Gain=Ki_y
  Kp_y : Gain  Gain=Kp_y
  Motor_Rwy : StateSpace  A=Arwy  B=Brwy  C=Crwy  D=Drwy  X0=Wy0
  Saturation : Saturate  UpperLimit=100  LowerLimit=-100
  Sum : Sum  Inputs=|+-
  Sum1 : Sum  Inputs=|++
  W_y : Outport
  cur_y : Outport  Port=2
  dW_y : Outport  Port=3
  wires:
  Sum/1 -> Ki_y/1, Kp_y/1
  Ki_y/1 -> Integrator/1
  Integrator/1 -> Sum1/2
  Kp_y/1 -> Sum1/1
  Sum1/1 -> Saturation/1
  Motor_Rwy/1 -> Demux/1
  Demux/1 -> Sum/2, W_y/1
  Saturation/1 -> Motor_Rwy/1
  Demux/2 -> cur_y/1
  Demux/3 -> dW_y/1
  Wy/1 -> Sum/1

== system Controle_UDP_0809_simulador/esfera /Rwz ==
  Wz : Inport
  Demux : Demux  Outputs=3
  Integrator : Integrator  InitialCondition=Wz0(1)/47.149
  Ki_z : Gain  Gain=Ki_z
  Kp_z : Gain  Gain=Kp_z
  Motor_Rwz : StateSpace  A=Arwz  B=Brwz  C=Crwz  D=Drwz  X0=Wz0
  Saturation : Saturate  UpperLimit=100  LowerLimit=-100
  Sum : Sum  Inputs=|+-
  Sum1 : Sum  Inputs=|++
  W_z : Outport
  cur_z : Outport  Port=2
  dW_z : Outport  Port=3
  wires:
  Saturation/1 -> Motor_Rwz/1
  Demux/1 -> Sum/2, W_z/1
  Demux/3 -> dW_z/1
  Motor_Rwz/1 -> Demux/1
  Sum1/1 -> Saturation/1
  Kp_z/1 -> Sum1/1
  Integrator/1 -> Sum1/2
  Ki_z/1 -> Integrator/1
  Sum/1 -> Ki_z/1, Kp_z/1
  Demux/2 -> cur_z/1
  Wz/1 -> Sum/1

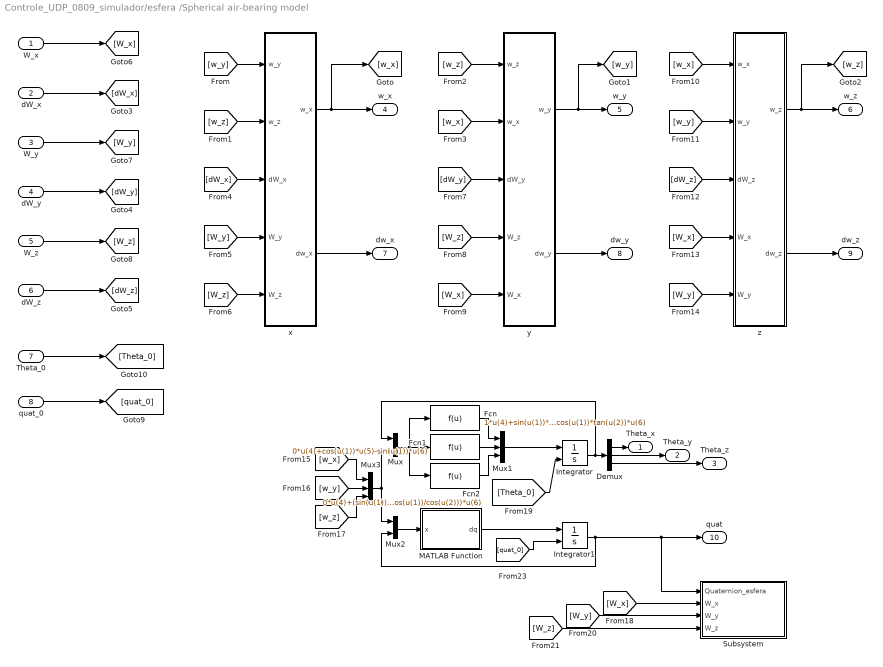
== system Controle_UDP_0809_simulador/esfera /Spherical air-bearing model ==
  W_x : Inport
  dW_x : Inport  Port=2
  W_y : Inport  Port=3
  dW_y : Inport  Port=4
  W_z : Inport  Port=5
  dW_z : Inport  Port=6
  Theta_0 : Inport  Port=7
  quat_0 : Inport  Port=8
  Demux : Demux  Outputs=3
  Fcn : Fcn  Expr=1*u(4)+sin(u(1))*tan(u(2))*u(5)+cos(u(1))*tan(u(2))*u(6)
  Fcn1 : Fcn  Expr=0*u(4)+cos(u(1))*u(5)-sin(u(1))*u(6)
  Fcn2 : Fcn  Expr=0*u(4)+(sin(u(1))/cos(u(2)))*u(5)+(cos(u(1))/cos(u(2)))*u(6)
  Integrator : Integrator  InitialConditionSource=external
  Integrator1 : Integrator  InitialConditionSource=external
  MATLAB Function : MATLAB Function  TreatAsAtomicUnit=on
  Mux : Mux  Inputs=2
  Mux1 : Mux  Inputs=3
  Mux2 : Mux  Inputs=2
  Mux3 : Mux  Inputs=3
  Subsystem : Subsystem
  x : Subsystem
      mask Display:
      | port_label('input',1,'\omega_{y}','texmode','on')
      | port_label('input',2,'\omega_{z}','texmode','on')
      | port_label('input',3,'d\Omega_{x}','texmode','on')
      | port_label('input',4,'\Omega_{y}','texmode','on')
      | port_label('input',5,'\Omega_{z}','texmode','on')
      | 
      | port_label('output',1,'\omega_x','texmode','on')
      | port_label('output',2,'d\omega_x','texmode','on')
  y : Subsystem
      mask Display:
      | port_label('input',1,'\omega_{z}','texmode','on')
      | port_label('input',2,'\omega_{x}','texmode','on')
      | port_label('input',3,'d\Omega_{y}','texmode','on')
      | port_label('input',4,'\Omega_{z}','texmode','on')
      | port_label('input',5,'\Omega_{x}','texmode','on')
      | 
      | port_label('output',1,'\omega_y','texmode','on')
      | port_label('output',2,'d\omega_y','texmode','on')
  z : Subsystem
      mask Display:
      | port_label('input',1,'\omega_{x}','texmode','on')
      | port_label('input',2,'\omega_{y}','texmode','on')
      | port_label('input',3,'d\Omega_{z}','texmode','on')
      | port_label('input',4,'\Omega_{x}','texmode','on')
      | port_label('input',5,'\Omega_{y}','texmode','on')
      | 
      | port_label('output',1,'\omega_z','texmode','on')
      | port_label('output',2,'d\omega_z','texmode','on')
  Theta_x : Outport
  Theta_y : Outport  Port=2
  Theta_z : Outport  Port=3
  w_x : Outport  Port=4
  w_y : Outport  Port=5
  w_z : Outport  Port=6
  dw_x : Outport  Port=7
  dw_y : Outport  Port=8
  dw_z : Outport  Port=9
  quat : Outport  Port=10
  wires:
  [w_y] -> x/1(w_y)
  [w_z] -> x/2(w_z)
  [dW_x] -> x/3(dW_x)
  dW_x/1 -> [dW_x]
  dW_y/1 -> [dW_y]
  dW_z/1 -> [dW_z]
  [W_y] -> x/4(W_y)
  [W_z] -> x/5(W_z)
  x/1(w_x) -> w_x/1, [w_x]
  x/2(dw_x) -> dw_x/1
  y/1(w_y) -> w_y/1, [w_y]
  y/2(dw_y) -> dw_y/1
  [w_z] -> y/1(w_z)
  [w_x] -> y/2(w_x)
  [dW_y] -> y/3(dW_y)
  [W_z] -> y/4(W_z)
  [W_x] -> y/5(W_x)
  [w_x] -> z/1(w_x)
  [w_y] -> z/2(w_y)
  [dW_z] -> z/3(dW_z)
  [W_x] -> z/4(W_x)
  [W_y] -> z/5(W_y)
  z/1(w_z) -> [w_z], w_z/1
  z/2(dw_z) -> dw_z/1
  W_x/1 -> [W_x]
  W_y/1 -> [W_y]
  W_z/1 -> [W_z]
  Integrator/1 -> Demux/1, Mux/1
  Mux1/1 -> Integrator/1
  Demux/1 -> Theta_x/1
  Demux/2 -> Theta_y/1
  Demux/3 -> Theta_z/1
  [Theta_0] -> Integrator/2
  Theta_0/1 -> [Theta_0]
  Fcn/1 -> Mux1/1
  Fcn1/1 -> Mux1/2
  Fcn2/1 -> Mux1/3
  Mux3/1 -> Mux/2, Mux2/1
  [w_x] -> Mux3/1
  [w_y] -> Mux3/2
  [w_z] -> Mux3/3
  Mux/1 -> Fcn1/1, Fcn2/1, Fcn/1
  Mux2/1 -> MATLAB Function/1(x)
  [quat_0] -> Integrator1/2
  MATLAB Function/1(dq) -> Integrator1/1
  quat_0/1 -> [quat_0]
  Integrator1/1 -> Mux2/2, quat/1, Subsystem/1(Quaternion_esfera)
  [W_x] -> Subsystem/2(W_x)
  [W_z] -> Subsystem/4(W_z)
  [W_y] -> Subsystem/3(W_y)

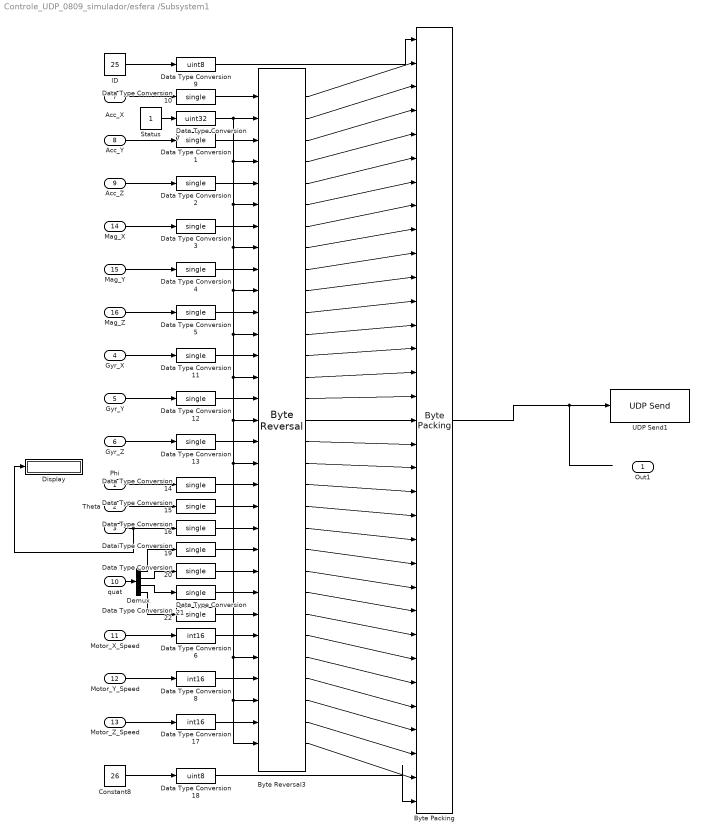
== system Controle_UDP_0809_simulador/esfera /Subsystem1 ==
  Phi : Inport
  Theta : Inport  Port=2
  Psi : Inport  Port=3
  Gyr_X : Inport  Port=4
  Gyr_Y : Inport  Port=5
  Gyr_Z : Inport  Port=6
  Acc_X : Inport  Port=7
  Acc_Y : Inport  Port=8
  Acc_Z : Inport  Port=9
  quat : Inport  Port=10
  Motor_X_Speed : Inport  Port=11
  Motor_Y_Speed : Inport  Port=12
  Motor_Z_Speed : Inport  Port=13
  Mag_X : Inport  Port=14
  Mag_Y : Inport  Port=15
  Mag_Z : Inport  Port=16
  "Byte Packing " : xpcutilitieslib/Byte Packing   MaskPackedDataType=uint8  MaskUnpackedDataTypes={'uint8','single','uint32','single', 'uint32', 'single', 'uint32', 'single', 'uint32', 'single', 'uint32', 'single', 'uint32', 'single', 'uint32', 'single', 'uint32', 'single', 'uint32', 'single', 'single', 'single','single','single','single','single', 'int16', 'uint32', 'int16', 'uint32', 'int16', 'uint32','uint8'}  MaskAlignment=1
  Byte Reversal3 : etargetslib/Byte Reversal  numInp=31
  Constant8 : Constant  Value=26  OutDataTypeStr=uint8
  Data Type Conversion{1..5,10..16,19..22} (16 alike) : DataTypeConversion  OutDataTypeStr=single  SaturateOnIntegerOverflow=on
  Data Type Conversion17 : DataTypeConversion  OutDataTypeStr=int16  SaturateOnIntegerOverflow=on
  Data Type Conversion18 : DataTypeConversion  OutDataTypeStr=uint8  SaturateOnIntegerOverflow=on
  Data Type Conversion6 : DataTypeConversion  OutDataTypeStr=int16  SaturateOnIntegerOverflow=on
  Data Type Conversion7 : DataTypeConversion  OutDataTypeStr=uint32  SaturateOnIntegerOverflow=on
  Data Type Conversion8 : DataTypeConversion  OutDataTypeStr=int16  SaturateOnIntegerOverflow=on
  Data Type Conversion9 : DataTypeConversion  OutDataTypeStr=uint8  SaturateOnIntegerOverflow=on
  Demux : Demux
  Display : Display
  ID : Constant  Value=25  OutDataTypeStr=uint8
  Status : Constant  OutDataTypeStr=uint32
  UDP Send1 : instrumentlib/UDP Send  Host=127.0.0.1  Port=35205  LocalPort=35204  EnableBlockingMode=off  ByteOrder=BigEndian
  Out1 : Outport
  wires:
  Constant8/1 -> Data Type Conversion18/1
  ID/1 -> Data Type Conversion9/1
  "Byte Packing "/1 -> UDP Send1/1
  Acc_X/1 -> Data Type Conversion10/1
  Acc_Z/1 -> Data Type Conversion2/1
  Mag_X/1 -> Data Type Conversion3/1
  Mag_Y/1 -> Data Type Conversion4/1
  Mag_Z/1 -> Data Type Conversion5/1
  Gyr_X/1 -> Data Type Conversion11/1
  Gyr_Y/1 -> Data Type Conversion12/1
  Gyr_Z/1 -> Data Type Conversion13/1
  Phi/1 -> Data Type Conversion14/1
  Theta/1 -> Data Type Conversion15/1
  Psi/1 -> Display/1, Data Type Conversion16/1
  Motor_Z_Speed/1 -> Data Type Conversion17/1
  Motor_Y_Speed/1 -> Data Type Conversion8/1
  Status/1 -> Data Type Conversion7/1
  Data Type Conversion10/1 -> Byte Reversal3/1
  Byte Reversal3/1 -> "Byte Packing "/2
  Byte Reversal3/3 -> "Byte Packing "/4
  Byte Reversal3/5 -> "Byte Packing "/6
  Byte Reversal3/7 -> "Byte Packing "/8
  Byte Reversal3/9 -> "Byte Packing "/10
  Byte Reversal3/11 -> "Byte Packing "/12
  Byte Reversal3/13 -> "Byte Packing "/14
  Byte Reversal3/15 -> "Byte Packing "/16
  Byte Reversal3/17 -> "Byte Packing "/18
  Byte Reversal3/19 -> "Byte Packing "/20
  Byte Reversal3/20 -> "Byte Packing "/21
  Byte Reversal3/21 -> "Byte Packing "/22
  Byte Reversal3/22 -> "Byte Packing "/23
  Byte Reversal3/2 -> "Byte Packing "/3
  Byte Reversal3/4 -> "Byte Packing "/5
  Byte Reversal3/6 -> "Byte Packing "/7
  Byte Reversal3/8 -> "Byte Packing "/9
  Byte Reversal3/10 -> "Byte Packing "/11
  Byte Reversal3/12 -> "Byte Packing "/13
  Byte Reversal3/14 -> "Byte Packing "/15
  Byte Reversal3/16 -> "Byte Packing "/17
  Byte Reversal3/18 -> "Byte Packing "/19
  Data Type Conversion2/1 -> Byte Reversal3/5
  Data Type Conversion3/1 -> Byte Reversal3/7
  Data Type Conversion4/1 -> Byte Reversal3/9
  Data Type Conversion5/1 -> Byte Reversal3/11
  Data Type Conversion11/1 -> Byte Reversal3/13
  Data Type Conversion12/1 -> Byte Reversal3/15
  Data Type Conversion13/1 -> Byte Reversal3/17
  Data Type Conversion14/1 -> Byte Reversal3/19
  Data Type Conversion15/1 -> Byte Reversal3/20
  Data Type Conversion16/1 -> Byte Reversal3/21
  Data Type Conversion19/1 -> Byte Reversal3/22
  Data Type Conversion8/1 -> Byte Reversal3/28
  Data Type Conversion17/1 -> Byte Reversal3/30
  Data Type Conversion6/1 -> Byte Reversal3/26
  Byte Reversal3/23 -> "Byte Packing "/24
  Byte Reversal3/24 -> "Byte Packing "/25
  Byte Reversal3/25 -> "Byte Packing "/26
  Byte Reversal3/26 -> "Byte Packing "/27
  Byte Reversal3/27 -> "Byte Packing "/28
  Byte Reversal3/28 -> "Byte Packing "/29
  Byte Reversal3/29 -> "Byte Packing "/30
  Byte Reversal3/30 -> "Byte Packing "/31
  Byte Reversal3/31 -> "Byte Packing "/32
  Data Type Conversion18/1 -> "Byte Packing "/33
  Data Type Conversion20/1 -> Byte Reversal3/23
  Data Type Conversion21/1 -> Byte Reversal3/24
  Data Type Conversion22/1 -> Byte Reversal3/25
  Motor_X_Speed/1 -> Data Type Conversion6/1
  Acc_Y/1 -> Data Type Conversion1/1
  Data Type Conversion1/1 -> Byte Reversal3/3
  Data Type Conversion7/1 -> Byte Reversal3/31, Byte Reversal3/29, Byte Reversal3/27, Byte Reversal3/18, Byte Reversal3/16, Byte Reversal3/14, Byte Reversal3/12, Byte Reversal3/10, Byte Reversal3/8, Byte Reversal3/6, Byte Reversal3/4, Byte Reversal3/2
  Data Type Conversion9/1 -> "Byte Packing "/1
  Demux/1 -> Data Type Conversion19/1
  Demux/2 -> Data Type Conversion20/1
  Demux/3 -> Data Type Conversion21/1
  Demux/4 -> Data Type Conversion22/1
  quat/1 -> Demux/1

== system Controle_UDP_0809_simulador/controle /Logica de controle/Gerador de sinal de referencia ==
  note: Referencias em graus!
  Gain3 : Gain  Gain=pi/180
  Mux5 : Mux  Inputs=3
  Referencia Pitch : simulink/Sources/Repeating Sequence Interpolated  OutValues=[0 0 5 5 -5 -5 0 0].'  TimeValues=[0 180 180.1 240 240.1 300 300.1 360].'  LookUpMeth=Interpolation-Use End Values  tsamp=-1  OutMin=[]  OutMax=[]  OutDataTypeStr=double  OutputDataTypeScalingMode=double  OutDataType=fixdt(0,8)  OutScaling=2^-10
  Referencia Roll : simulink/Sources/Repeating Sequence Interpolated  OutValues=[5 5 -5 -5 0 0].'  TimeValues=[0 60 60.1 120 120.1 360].'  LookUpMeth=Interpolation-Use End Values  tsamp=-1  OutMin=[]  OutMax=[]  OutDataTypeStr=double  OutputDataTypeScalingMode=double  OutDataType=fixdt(0,8)  OutScaling=2^-10
  Referencia Yaw : simulink/Sources/Repeating Sequence Interpolated  OutValues=[0 0 0 0 0].'  TimeValues=[0 0.1 0.5 0.6 1].'  LookUpMeth=Interpolation-Use End Values  tsamp=-1  OutMin=[]  OutMax=[]  OutDataTypeStr=double  OutputDataTypeScalingMode=double  OutDataType=fixdt(0,8)  OutScaling=2^-10
  Out1 : Outport
  wires:
  Referencia Pitch/1 -> Mux5/2
  Mux5/1 -> Gain3/1
  Referencia Yaw/1 -> Mux5/3
  Referencia Roll/1 -> Mux5/1
  Gain3/1 -> Out1/1

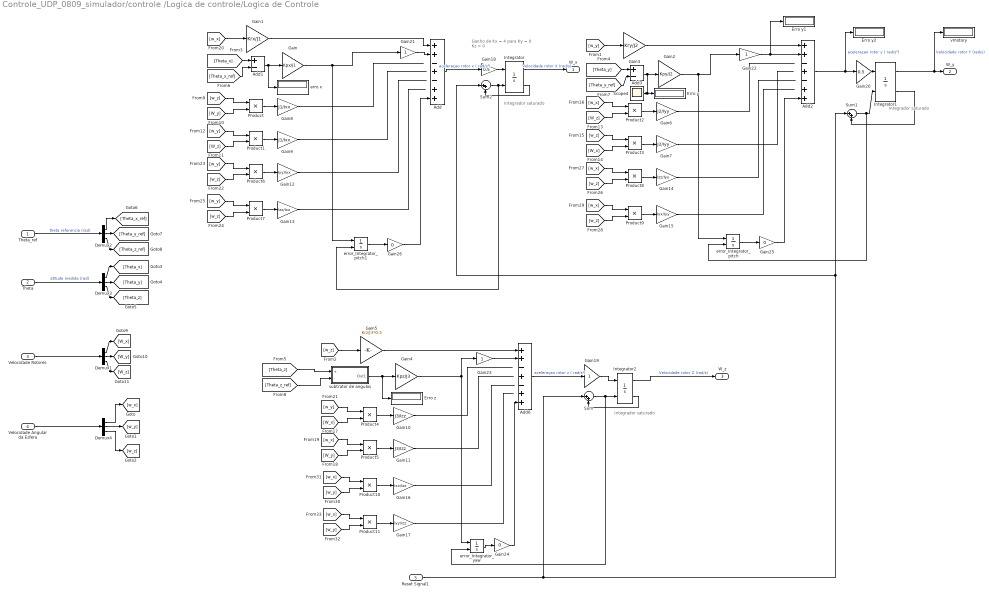
== system Controle_UDP_0809_simulador/controle /Logica de controle/Logica de Controle ==
  note: Ganho de Kx = 4
      | para Ky = 0
      | Kz = 0
  note: Integrador
      | saturado
  note: Integrador
      | saturado
  note: Integrador
      | saturado
  Theta_ref : Inport
  Theta : Inport  Port=2
  Velocidade Rotores : Inport  Port=3
  Velocidade Angular da Esfera : Inport  Port=4
  Reset Signal1 : Inport  Port=5
  Add : Sum  Inputs=++-+-++
  Add1 : Sum  Inputs=+-
  Add2 : Sum  Inputs=++-+-++
  Add3 : Sum  Inputs=+-
  Add6 : Sum  Inputs=++-+-++
  Demux{1..4} (4 alike) : Demux  Outputs=3
  Erro y : Display
  Erro y1 : Display
  Erro y2 : Display
  Erro z : Display
  Gain : Gain  Gain=Kpx/J1
  Gain1 : Gain  Gain=Krx/J1
  Gain10 : Gain  Gain=J3/Izz
  Gain11 : Gain  Gain=J3/Izz
  Gain12 : Gain  Gain=Iyy/Ixx
  Gain13 : Gain  Gain=Izz/Ixx
  Gain14 : Gain  Gain=Izz/Iyy
  Gain15 : Gain  Gain=Ixx/Iyy
  Gain16 : Gain  Gain=Ixx/Izz
  Gain17 : Gain  Gain=Iyy/Izz
  Gain18 : Gain  Gain=0.5  SaturateOnIntegerOverflow=on
  Gain{19,21..23} (4 alike) : Gain  SaturateOnIntegerOverflow=on
  Gain2 : Gain  Gain=Kpy/J2
  Gain20 : Gain  Gain=0.5  SaturateOnIntegerOverflow=on
  Gain24 : Gain  Gain=0  SaturateOnIntegerOverflow=on
  Gain25 : Gain  Gain=0  SaturateOnIntegerOverflow=on
  Gain26 : Gain  Gain=0  SaturateOnIntegerOverflow=on
  Gain3 : Gain  Gain=Kry/J2
  Gain4 : Gain  Gain=Kpz/J3
  Gain5 : Gain  Gain=Krz/J3*0.5
  Gain6 : Gain  Gain=J2/Iyy
  Gain7 : Gain  Gain=J2/Iyy
  Gain8 : Gain  Gain=J1/Ixx
  Gain9 : Gain  Gain=J1/Ixx
  Integrator : Integrator  ExternalReset=level  InitialCondition=Wx0(1)  LimitOutput=on  UpperSaturationLimit=Wx0(1)+4000*2*pi/60  LowerSaturationLimit=Wx0(1)-4000*2*pi/60  ShowSaturationPort=on
  Integrator1 : Integrator  ExternalReset=level  InitialCondition=Wy0(1)  LimitOutput=on  UpperSaturationLimit=Wy0(1)+4000*2*pi/60  LowerSaturationLimit=Wy0(1)-4000*2*pi/60  ShowSaturationPort=on
  Integrator2 : Integrator  ExternalReset=level  InitialCondition=Wz0(1)  LimitOutput=on  UpperSaturationLimit=Wz0(1)+4000*2*pi/60  LowerSaturationLimit=Wz0(1)-4000*2*pi/60  ShowSaturationPort=on
  Product{,1..11} (12 alike) : Product  RndMeth=Zero
  Scope4 : Scope
      settings: TimeRange=2  YMin=-0.35  YMax=0  SaveName=ScopeData5
  Sum : Sum  Inputs=|++  AccumDataTypeStr=double  OutDataTypeStr=double
  Sum1 : Sum  Inputs=|++  OutDataTypeStr=double
  Sum2 : Sum  Inputs=|++  OutDataTypeStr=double
  erro x : Display
  error_Integrator_pitch : Integrator  ExternalReset=level
  error_Integrator_pitch1 : Integrator  ExternalReset=level
  error_Integrator_yaw : Integrator  ExternalReset=level
  subtrator de angulos : Subsystem
  vmotory : Display
  W_x : Outport
  W_y : Outport  Port=2
  W_z : Outport  Port=3
  wires:
  [w_x] -> Gain1/1
  Add1/1 -> Gain/1, erro x/1
  [w_y] -> Gain3/1
  Add3/1 -> Gain2/1, Scope4/1, Erro y/1
  [w_z] -> Gain5/1
  Add2/1 -> Erro y2/1, Gain20/1  "aceleraçao rotor y ( rad/s²)"
  Gain/1 -> error_Integrator_pitch1/1, Gain21/1
  [Theta_x] -> Add1/1
  [Theta_x_ref] -> Add1/2
  Gain2/1 -> error_Integrator_pitch/1, Gain22/1
  Gain3/1 -> Add2/1
  [Theta_y] -> Add3/1
  [Theta_y_ref] -> Add3/2
  Gain5/1 -> Add6/1
  [Theta_z] -> subtrator de angulos/1(+)
  [Theta_z_ref] -> subtrator de angulos/2(-)
  Velocidade Rotores/1 -> Demux1/1
  Theta_ref/1 -> Demux2/1  "theta referencia (rad)"
  Demux1/1 -> [W_x]
  Demux1/2 -> [W_y]
  Demux1/3 -> [W_z]
  Demux3/1 -> [Theta_x]
  Demux3/2 -> [Theta_y]
  Demux3/3 -> [Theta_z]
  Demux2/1 -> [Theta_x_ref]
  Demux2/2 -> [Theta_y_ref]
  Demux2/3 -> [Theta_z_ref]
  [w_z] -> Product/1
  [W_y] -> Product/2
  Product/1 -> Gain8/1
  [w_y] -> Product1/1
  [W_z] -> Product1/2
  Product1/1 -> Gain9/1
  [w_x] -> Product2/1
  [W_z] -> Product2/2
  Product2/1 -> Gain6/1
  [w_z] -> Product3/1
  [W_x] -> Product3/2
  Product3/1 -> Gain7/1
  [w_y] -> Product4/1
  [W_x] -> Product4/2
  Product4/1 -> Gain10/1
  [w_x] -> Product5/1
  [W_y] -> Product5/2
  Product5/1 -> Gain11/1
  Gain6/1 -> ?
  Gain7/1 -> ?
  Gain8/1 -> ?
  Gain9/1 -> ?
  [w_y] -> Product6/1
  [w_z] -> Product6/2
  Product6/1 -> Gain12/1
  Gain12/1 -> ?
  [w_y] -> Product7/1
  [w_z] -> Product7/2
  Product7/1 -> Gain13/1
  [w_x] -> Product8/1
  [w_z] -> Product8/2
  Product8/1 -> Gain14/1
  [w_x] -> Product9/1
  [w_z] -> Product9/2
  Product9/1 -> Gain15/1
  Gain14/1 -> ?
  Gain15/1 -> ?
  [w_x] -> Product10/1
  [w_y] -> Product10/2
  Product10/1 -> Gain16/1
  [w_x] -> Product11/1
  [w_y] -> Product11/2
  Product11/1 -> Gain17/1
  Gain10/1 -> ?
  Gain11/1 -> ?
  Gain16/1 -> ?
  Gain17/1 -> ?
  Add6/1 -> Gain19/1  "aceleraçao rotor z ( rad/s²)"
  Gain13/1 -> ?
  Add/1 -> Gain18/1  "aceleraçao rotor x ( rad/s²)"
  subtrator de angulos/1(Out1) -> Erro z/1, Gain4/1
  Integrator/1 -> W_x/1  "Velocidade rotor X (rad/s)"
  Integrator2/1 -> W_z/1  "Velocidade rotor Z (rad/s)"
  Integrator1/1 -> vmotory/1, W_y/1  "Velocidade rotor Y (rad/s)"
  Theta/1 -> Demux3/1  "atitude medida (rad)"
  Reset Signal1/1 -> Sum/1, Sum2/1, Sum1/1
  Gain19/1 -> Integrator2/1
  Gain20/1 -> Integrator1/1
  Gain18/1 -> Integrator/1
  Velocidade Angular da Esfera/1 -> Demux4/1
  Demux4/2 -> [w_y]
  Demux4/1 -> [w_x]
  Demux4/3 -> [w_z]
  Gain1/1 -> Add/1
  Gain21/1 -> Add/2
  Gain22/1 -> Erro y1/1, Add2/2
  Gain23/1 -> Add6/2
  error_Integrator_pitch/1 -> Gain25/1
  Gain25/1 -> Add2/7
  Integrator2/2 -> Sum/2
  Sum/1 -> error_Integrator_yaw/2, Integrator2/2
  Gain4/1 -> Gain23/1, error_Integrator_yaw/1
  error_Integrator_yaw/1 -> Gain24/1
  Gain24/1 -> Add6/7
  Integrator1/2 -> Sum1/2
  Sum1/1 -> Integrator1/2, error_Integrator_pitch/2
  Integrator/2 -> Sum2/2
  Sum2/1 -> error_Integrator_pitch1/2, Integrator/2
  error_Integrator_pitch1/1 -> Gain26/1
  Gain26/1 -> Add/7
